simulink model "branchmodel"  (R2026a)
settings: Solver=VariableStepAuto  StopTime=480
undefined symbols (not defined in the file): exprnd, m, n
settings Model: Creator=Sayandip Mallick  LastModifiedBy=Sayandip Mallick

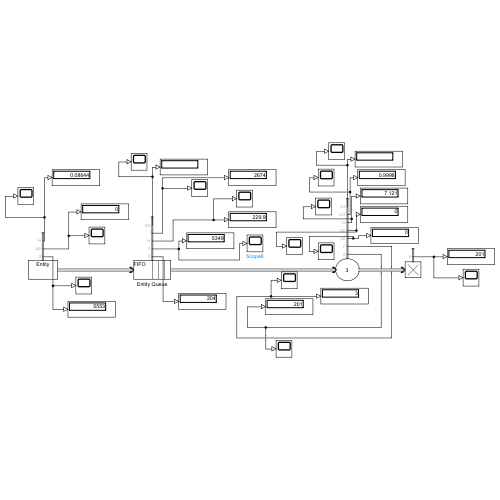
[thumbnail: Simulink's stored preview of the top-level diagram]
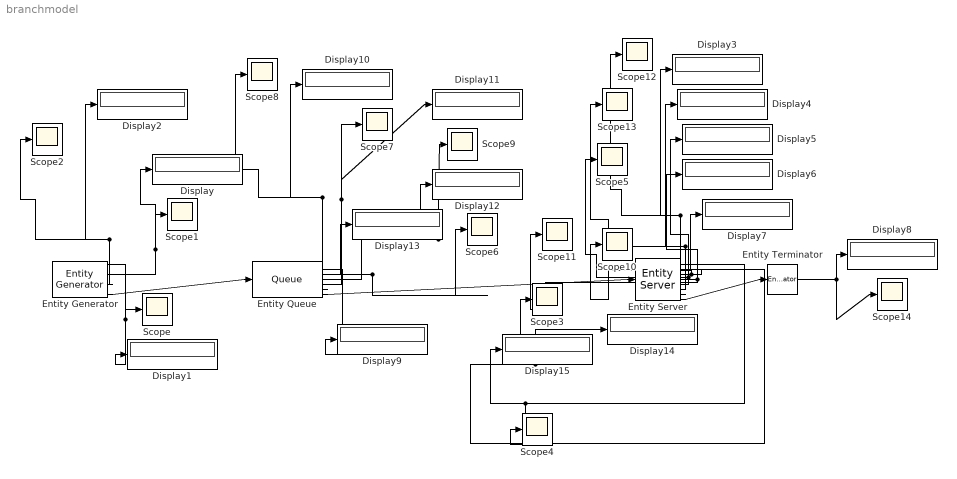
== system branchmodel ==
  Display{,1..15} (16 alike) : Display
  Entity Generator : EntityGenerator  OutputPortMessageModes=n,n,n,m  Period=exprnd(2)  AttributeName=Patience  AttributeInitialValue=exprnd(15)  NumberEntitiesDeparted=on  PendingEntityInBlock=on  AverageIntergenerationTime=on  EntityType=Structured  EntityTypeName=Entity
      settings: OutputPortMap=o0,o1,o2,o3
  Entity Queue : Queue  InputPortMessageModes=m  OutputPortMessageModes=n,n,n,n,n,m  Capacity=inf  NumberEntitiesDeparted=on  NumEntitiesExtracted=on  NumberEntitiesInBlock=on  AverageWait=on  AverageQueueLength=on
      settings: OutputPortMap=o0,o1,o2,o3,o7,o5
  Entity Server : EntityServer  InputPortMessageModes=m  OutputPortMessageModes=n,n,n,n,n,n,n,m  Capacity=3  ServiceTimeValue=exprnd(5)  NumberEntitiesDeparted=on  NumberEntitiesInBlock=on  PendingEntityPresentInBlock=on  NumberEntitiesPending=on  AverageWait=on  Utilization=on  NumEntitiesExtracted=on
      settings: OutputPortMap=o0,o1,o2,o3,o4,o5,o12,o9
  Entity Terminator : EntityTerminator  InputPortMessageModes=m  NumberEntitiesArrived=on
      settings: OutputPortMap=o0
  Scope{,1..14} (15 alike) : Scope
      Scope settings: ActiveDisplayYMinimum=-27.7278440323773  ActiveDisplayYMaximum=110.22229168007505
      Scope1 settings: ActiveDisplayYMinimum=-4.9432312613136791  ActiveDisplayYMaximum=4.0571883619976372
      Scope10 settings: DataLoggingVariableName=ScopeData10
      Scope11 settings: DataLoggingVariableName=ScopeData11
      Scope12 settings: DataLoggingVariableName=ScopeData12
      Scope13 settings: DataLoggingVariableName=ScopeData13
      Scope14 settings: ActiveDisplayYMinimum=-20.662925191651141  ActiveDisplayYMaximum=117.60091074584892  DataLoggingVariableName=ScopeData14
      Scope2 settings: ActiveDisplayYMinimum=-6.7128434919080711  ActiveDisplayYMaximum=83.510693955675961  DataLoggingVariableName=ScopeData2
      Scope3 settings: DataLoggingVariableName=ScopeData3
      Scope4 settings: DataLoggingVariableName=ScopeData4
      Scope5 settings: ActiveDisplayYMinimum=1.2328024708004028  ActiveDisplayYMaximum=1.7773948519413065  DataLoggingVariableName=ScopeData5
      Scope6 settings: ActiveDisplayYMinimum=-810.37384822604963  ActiveDisplayYMaximum=4995.18787833645  DataLoggingVariableName=ScopeData6
      Scope7 settings: DataLoggingVariableName=ScopeData7
      Scope8 settings: DataLoggingVariableName=ScopeData8
      Scope9 settings: ActiveDisplayYMinimum=13.230435439109669  ActiveDisplayYMaximum=22.958209228904579  DataLoggingVariableName=ScopeData9
  wires:
  Entity Generator/4 -> Entity Queue/1
  Entity Queue/6 -> Entity Server/1
  Entity Server/8 -> Entity Terminator/1
  Entity Terminator/1 -> Scope14/1, Display8/1
  Entity Server/2 -> Scope3/1, Display14/1
  Entity Server/1 -> Scope4/1, Display15/1
  Entity Generator/2 -> Scope1/1, Display/1
  Entity Generator/1 -> Scope/1, Display1/1
  Entity Generator/3 -> Display2/1, Scope2/1
  Entity Server/7 -> Display3/1, Scope12/1
  Entity Server/6 -> Display4/1, Scope13/1
  Entity Server/5 -> Scope5/1, Display5/1
  Entity Server/4 -> Display6/1, Scope11/1
  Entity Server/3 -> Scope10/1, Display7/1
  Entity Queue/1 -> Display9/1
  Entity Queue/5 -> Scope8/1, Display10/1
  Entity Queue/4 -> Scope7/1, Display11/1
  Entity Queue/3 -> Scope9/1, Display12/1
  Entity Queue/2 -> Scope6/1, Display13/1
